simulink model "RLC_model_2_input_finder"  (R2022a)
settings: Solver=FixedStepAuto  StartTime=0.0  StopTime=.004  FixedStep=1e-7  RelTol=1e-3
model workspace (MAT data in the model file):
  Amplitude = 1800
values from neighbouring files (symbols this model uses):
  Amp = Amplitude    [RLC_input_finder.m]
  frequency = round(double(frequency))    [RLC_Square_Wave_Driver.m]    (also in RLC_input_finder.m = i; Voltage_Waveform_Generator.m = 19000)
libraries: spsSeriesRLCBranchLib x15, spsVoltageMeasurementLib x5, simulink x3, spsControlledVoltageSourceLib x3, spsCurrentMeasurementLib x3, spsParallelRLCBranchLib x3, spsACCurrentSourceLib x1, spspowerguiLib x1
settings Model: Creator=ducks  LastModifiedBy=ducks

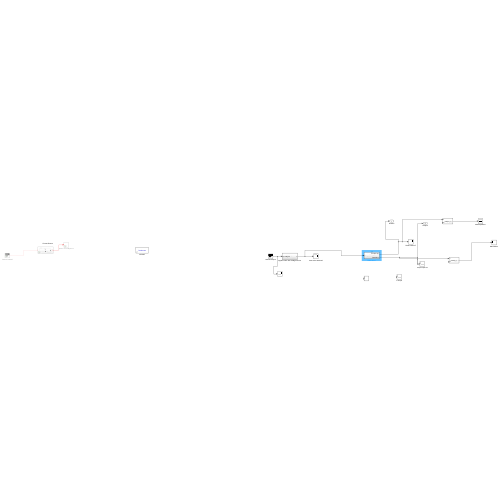
[thumbnail: Simulink's stored preview of the top-level diagram]
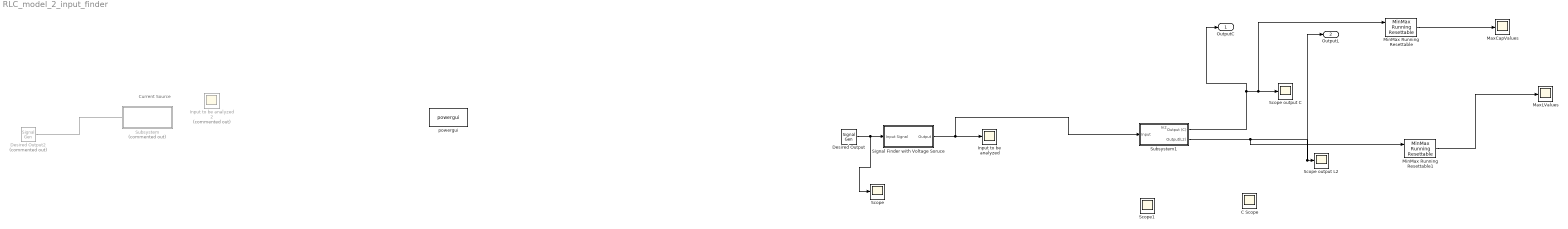
== system RLC_model_2_input_finder ==
  note: Current Source
  C Scope : Scope
  Desired Output : SignalGenerator  Amplitude=Amp  Frequency=frequency
  Desired Output2 : SignalGenerator  Commented=on  Amplitude=10000  Frequency=19100
  Input to be analyzed : Scope
  Input to be analyzed 2 : Scope  Commented=on
  MaxCapValues : Scope
  MaxLValues : Scope
  MinMax Running Resettable : simulink/Math Operations/MinMax Running Resettable  Function=max  vinit=0.0
  MinMax Running Resettable1 : simulink/Math Operations/MinMax Running Resettable  Function=max  vinit=0.0
  Scope : Scope
  Scope output C : Scope
  Scope output L2 : Scope
  Scope1 : Scope
  Signal Finder with Voltage Soruce : Subsystem
  Subsystem : Subsystem  Commented=on
  Subsystem1 : Subsystem
      settings: PortSchema="{\"entries\":[{\"content\":{\"sides\":[{\"content\":{\"connectorIds\":[\"In1\"]},\"type\":\"ConnectorPlacement.EquallySpacedRectSide\",\"uuid\":\"875611cf-7eb9-4d9d-822a-bd3f6d836b83\"},{\"content\":{\"connectorIds\":[\"Out1\",\"Out2\"],\"side\":\"RIGHT\"},\"type\":\"ConnectorPlacement.EquallySpacedRectSide\",\"uuid\":\"445ca6a9-d919-4b8d-ac4c-5af6ec8f882d\"},{\"content\":{\"connectorIds\":[\"In2\"],\"side\":\"TOP\"},\"type\":\"ConnectorPlacement.EquallySpacedRectSide\",\"uuid\":\"dd4cb797-8dc0-482e-83b9-0fae008e5cb7\"}]},\"type\":\"ConnectorPlacement.EquallySpacedConnector\",\"uuid\":\"ab642c4d-046c-490f-ad99-85f64f30cc72\"}],\"packageUris\":[\"http://schema.mathworks.com/mf0/Connector/R2020b\"],\"version\":\"1.0\"}"
  powergui : spspowerguiLib/powergui  Priority=1  SimulationMode=Continuous  SampleTime=50e-6  frequency=60  Iterations=50  frequencyindice=0  Pbase=100e6  ErrMax=1e-4  UnitsV=kV  UnitsW=MW  buscounter=0  FunctionMessages=off  echomessages=off  EnableUseOfTLC=off  CurrentSourceSwitches=off  DisableSnubberDevices=off  DisableRonSwitches=off  DisableVfSwitches=off  DisplayEquations=off  AutomaticDiscreteSolvers=off  SolverType=Tustin/Backward Euler (TBE)  Interpol=off  ExternalGateDelay=off  methode=off  Ts=100  x0status=blocks  SPID=on  SwTol=0  HookPort=off  NonlinearTolerance=1e-4  nMaxIteration=100  ContinueOnMaxIteration=off  RestoreLinks=warning  ResistiveCurrentMeasurement=off  Frange=[0:2:500]  Ylog=off  Xlog=on  ShowGrid=off  save=off  variable=ZData  structure=0  ZoomFFT=off  StartTime=0.0  cycles=1  DisplayStyle=1  fundamental=60  FreqAxis=off  MaxFrequency=1000  frequencyindicesteady=1  RmsSteady=1  display=off
  OutputC : Outport
  OutputL : Outport  Port=2
  wires:
  Desired Output2/1 -> ?
  ? -> Input to be analyzed 2/1
  Subsystem1/2(Output(L2)) -> MinMax Running Resettable1/1, OutputL/1, Scope output L2/1
  MinMax Running Resettable1/1 -> MaxLValues/1
  Desired Output/1 -> Scope/1, Signal Finder with Voltage Soruce/1(Input Signal)
  MinMax Running Resettable/1 -> MaxCapValues/1
  Subsystem1/1(Output (C)) -> OutputC/1, MinMax Running Resettable/1, Scope output C/1
  Signal Finder with Voltage Soruce/1(Output) -> Subsystem1/1(Input), Input to be analyzed/1

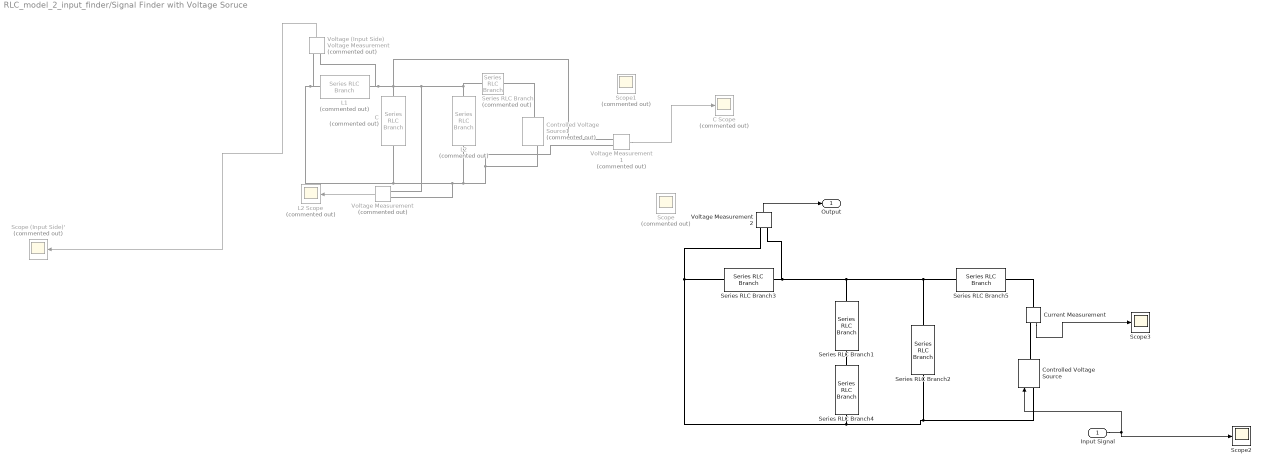
== system RLC_model_2_input_finder/Signal Finder with Voltage Soruce ==
  Input Signal : Inport
  C : spsSeriesRLCBranchLib/Series RLC Branch  Commented=on  LConnTagsString=__new0  RConnTagsString=__new0  BranchType=C  Resistance=1  Inductance=1e-3  SetiL0=off  InitialCurrent=0  Capacitance=96e-6  Setx0=off  InitialVoltage=0  Measurements=None
  C Scope : Scope  Commented=on
  Controlled Voltage Source : spsControlledVoltageSourceLib/Controlled Voltage Source  Initialize=on  Source_Type=AC  Amplitude=0  Phase=0  Frequency=0  Measurements=None
  Controlled Voltage Source1 : spsControlledVoltageSourceLib/Controlled Voltage Source  Commented=on  Initialize=on  Source_Type=DC  Amplitude=5  Phase=0  Frequency=0  Measurements=None
  Current Measurement : spsCurrentMeasurementLib/Current Measurement  PhasorSimulation=off  OutputType=Complex  PSBequivalent=0
  L1 : spsSeriesRLCBranchLib/Series RLC Branch  Commented=on  LConnTagsString=__new0  RConnTagsString=__new0  BranchType=L  Resistance=1  Inductance=1.4e-6  SetiL0=off  InitialCurrent=0  Capacitance=0  Setx0=off  InitialVoltage=0  Measurements=None
  L2 : spsSeriesRLCBranchLib/Series RLC Branch  Commented=on  LConnTagsString=__new0  RConnTagsString=__new0  BranchType=L  Resistance=1  Inductance=1.5e-6  SetiL0=off  InitialCurrent=0  Capacitance=1e-6  Setx0=off  InitialVoltage=0  Measurements=None
  L2 Scope : Scope  Commented=on
  Scope : Scope  Commented=on
  Scope (Input Side)' : Scope  Commented=on
  Scope1 : Scope  Commented=on
  Scope2 : Scope
  Scope3 : Scope
  Series RLC Branch : spsSeriesRLCBranchLib/Series RLC Branch  Commented=on  LConnTagsString=__new0  RConnTagsString=__new0  BranchType=R  Resistance=.001  Inductance=1e-3  SetiL0=off  InitialCurrent=0  Capacitance=1e-6  Setx0=off  InitialVoltage=0  Measurements=None
  Series RLC Branch1 : spsSeriesRLCBranchLib/Series RLC Branch  LConnTagsString=__new0  RConnTagsString=__new0  BranchType=C  Resistance=1  Inductance=1e-3  SetiL0=off  InitialCurrent=0  Capacitance=96e-6  Setx0=off  InitialVoltage=0  Measurements=None
  Series RLC Branch2 : spsSeriesRLCBranchLib/Series RLC Branch  LConnTagsString=__new0  RConnTagsString=__new0  BranchType=L  Resistance=1  Inductance=1.5e-6  SetiL0=off  InitialCurrent=0  Capacitance=1e-6  Setx0=off  InitialVoltage=0  Measurements=None
  Series RLC Branch3 : spsSeriesRLCBranchLib/Series RLC Branch  LConnTagsString=__new0  RConnTagsString=__new0  BranchType=L  Resistance=1  Inductance=1.4e-6  SetiL0=off  InitialCurrent=0  Capacitance=1e-6  Setx0=off  InitialVoltage=0  Measurements=None
  Series RLC Branch4 : spsSeriesRLCBranchLib/Series RLC Branch  LConnTagsString=__new0  RConnTagsString=__new0  BranchType=R  Resistance=.00159  Inductance=1e-3  SetiL0=off  InitialCurrent=0  Capacitance=1e-6  Setx0=off  InitialVoltage=0  Measurements=None
  Series RLC Branch5 : spsSeriesRLCBranchLib/Series RLC Branch  LConnTagsString=__new0  RConnTagsString=__new0  BranchType=R  Resistance=.01  Inductance=1e-3  SetiL0=off  InitialCurrent=0  Capacitance=1e-6  Setx0=off  InitialVoltage=0  Measurements=None
  Voltage (Input Side) : spsVoltageMeasurementLib/Voltage Measurement  Commented=on  PhasorSimulation=off  OutputType=Complex  PSBequivalent=0
  Voltage Measurement : spsVoltageMeasurementLib/Voltage Measurement  Commented=on  PhasorSimulation=off  OutputType=Complex  PSBequivalent=0
  Voltage Measurement1 : spsVoltageMeasurementLib/Voltage Measurement  Commented=on  PhasorSimulation=off  OutputType=Complex  PSBequivalent=0
  Voltage Measurement2 : spsVoltageMeasurementLib/Voltage Measurement  PhasorSimulation=off  OutputType=Complex  PSBequivalent=0
  Output : Outport
  wires:
  Voltage Measurement/1 -> L2 Scope/1
  Voltage (Input Side)/1 -> Scope (Input Side)'/1
  Voltage Measurement1/1 -> C Scope/1
  Input Signal/1 -> Controlled Voltage Source/1, Scope2/1
  Current Measurement/1 -> Scope3/1
  Voltage Measurement2/1 -> Output/1
  connections:
  Voltage Measurement1/LConn1 -- Series RLC Branch/LConn1 -- L2/LConn1 -- Voltage Measurement/LConn2 -- Voltage (Input Side)/LConn2 -- L1/RConn1 -- C/LConn1
  Controlled Voltage Source1/LConn1 -- Voltage Measurement1/LConn2 -- L2/RConn1 -- C/RConn1 -- Voltage (Input Side)/LConn1 -- L1/LConn1 -- Voltage Measurement/LConn1
  Series RLC Branch/RConn1 -- Controlled Voltage Source1/RConn1
  Controlled Voltage Source/LConn1 -- Series RLC Branch4/RConn1 -- Series RLC Branch3/LConn1 -- Voltage Measurement2/LConn1 -- Series RLC Branch2/RConn1
  Current Measurement/RConn1 -- Controlled Voltage Source/RConn1
  Series RLC Branch3/RConn1 -- Series RLC Branch5/LConn1 -- Series RLC Branch2/LConn1 -- Series RLC Branch1/LConn1 -- Voltage Measurement2/LConn2
  Series RLC Branch4/LConn1 -- Series RLC Branch1/RConn1
  Series RLC Branch5/RConn1 -- Current Measurement/LConn1

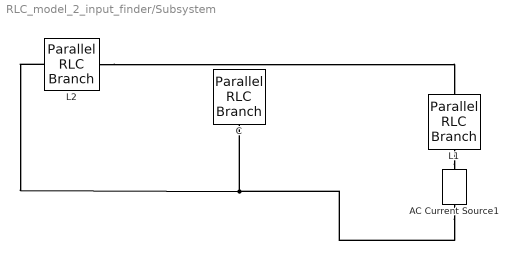
== system RLC_model_2_input_finder/Subsystem ==
  AC Current Source1 : spsACCurrentSourceLib/AC Current Source  Amplitude=1800  Phase=0  Frequency=19500  SampleTime=0  Measurements=None
      settings: SourceProductBaseCode=PS
  C : spsParallelRLCBranchLib/Parallel RLC Branch  LConnTagsString=a  RConnTagsString=__new0  BranchType=C  Resistance=1  Inductance=1e-3  SetiL0=off  InitialCurrent=0  Capacitance=96e-6  Setx0=off  InitialVoltage=0  Measurements=None
  L1 : spsParallelRLCBranchLib/Parallel RLC Branch  LConnTagsString=a  RConnTagsString=__new0  BranchType=L  Resistance=1  Inductance=2e-6  SetiL0=off  InitialCurrent=0  Capacitance=1e-6  Setx0=off  InitialVoltage=0  Measurements=None
  L2 : spsParallelRLCBranchLib/Parallel RLC Branch  LConnTagsString=a  RConnTagsString=__new0  BranchType=L  Resistance=1  Inductance=10e-6  SetiL0=off  InitialCurrent=0  Capacitance=1e-6  Setx0=off  InitialVoltage=0  Measurements=None
  connections:
  L2/RConn1 -- L1/LConn1
  L1/RConn1 -- AC Current Source1/RConn1
  AC Current Source1/LConn1 -- C/RConn1 -- L2/LConn1

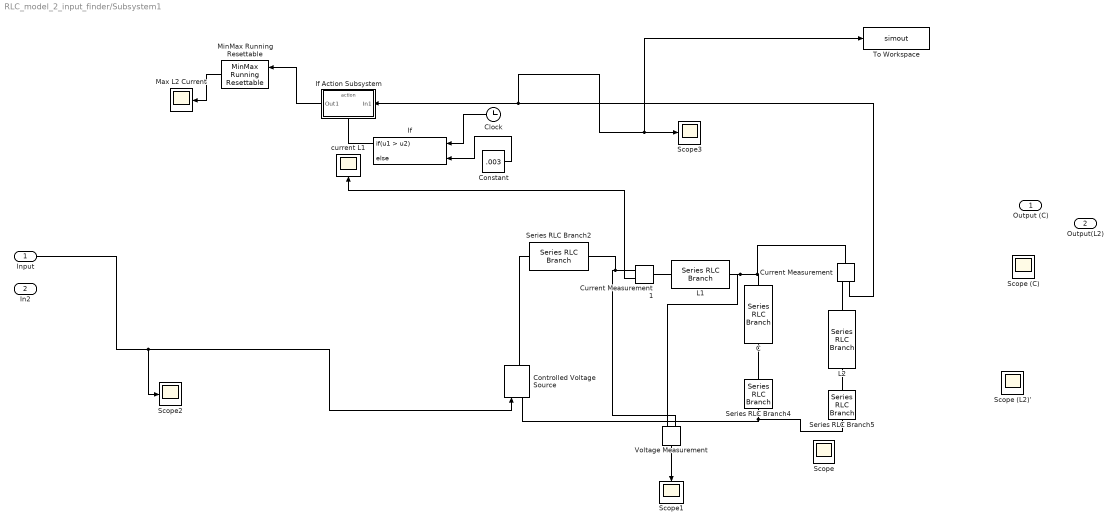
== system RLC_model_2_input_finder/Subsystem1 ==
  Input : Inport
  In2 : Inport  Port=2
  C : spsSeriesRLCBranchLib/Series RLC Branch  LConnTagsString=__new0  RConnTagsString=__new0  BranchType=C  Resistance=1  Inductance=1e-3  SetiL0=off  InitialCurrent=0  Capacitance=96e-6  Setx0=off  InitialVoltage=0  Measurements=None
  Clock : Clock
  Constant : Constant  Value=.003
  Controlled Voltage Source : spsControlledVoltageSourceLib/Controlled Voltage Source  Initialize=on  Source_Type=AC  Amplitude=0  Phase=0  Frequency=0  Measurements=None
  Current Measurement : spsCurrentMeasurementLib/Current Measurement  PhasorSimulation=off  OutputType=Complex  PSBequivalent=0
  Current Measurement1 : spsCurrentMeasurementLib/Current Measurement  PhasorSimulation=off  OutputType=Complex  PSBequivalent=0
  If : If  NumInputs=2  IfExpression=u1 > u2
  If Action Subsystem : Subsystem  TreatAsAtomicUnit=on
  L1 : spsSeriesRLCBranchLib/Series RLC Branch  LConnTagsString=__new0  RConnTagsString=__new0  BranchType=L  Resistance=1  Inductance=1.4e-6  SetiL0=off  InitialCurrent=0  Capacitance=0  Setx0=off  InitialVoltage=0  Measurements=None
  L2 : spsSeriesRLCBranchLib/Series RLC Branch  LConnTagsString=__new0  RConnTagsString=__new0  BranchType=L  Resistance=1  Inductance=1.5e-6  SetiL0=off  InitialCurrent=0  Capacitance=1e-6  Setx0=off  InitialVoltage=0  Measurements=None
  Max L2 Current : Scope
  MinMax Running Resettable : simulink/Math Operations/MinMax Running Resettable  Function=max  vinit=0.0
  Scope{,1..3} (4 alike) : Scope
  Scope (C) : Scope
  Scope (L2)' : Scope
  Series RLC Branch2 : spsSeriesRLCBranchLib/Series RLC Branch  LConnTagsString=__new0  RConnTagsString=__new0  BranchType=R  Resistance=.00164  Inductance=1e-3  SetiL0=off  InitialCurrent=0  Capacitance=1e-6  Setx0=off  InitialVoltage=0  Measurements=None
  Series RLC Branch4 : spsSeriesRLCBranchLib/Series RLC Branch  LConnTagsString=__new0  RConnTagsString=__new0  BranchType=R  Resistance=.00205  Inductance=1e-3  SetiL0=off  InitialCurrent=0  Capacitance=1e-6  Setx0=off  InitialVoltage=0  Measurements=None
  Series RLC Branch5 : spsSeriesRLCBranchLib/Series RLC Branch  LConnTagsString=__new0  RConnTagsString=__new0  BranchType=R  Resistance=.00205  Inductance=1e-3  SetiL0=off  InitialCurrent=0  Capacitance=1e-6  Setx0=off  InitialVoltage=0  Measurements=None
  To Workspace : ToWorkspace  VariableName=simout  SaveFormat=Timeseries  SampleTime=-1
  Voltage Measurement : spsVoltageMeasurementLib/Voltage Measurement  PhasorSimulation=off  OutputType=Complex  PSBequivalent=0
  current L1 : Scope
  Output (C) : Outport
  Output(L2) : Outport  Port=2
  wires:
  Voltage Measurement/1 -> Scope1/1
  Input/1 -> Scope2/1, Controlled Voltage Source/1
  Current Measurement/1 -> If Action Subsystem/1(In1), To Workspace/1, Scope3/1
  Current Measurement1/1 -> current L1/1
  Clock/1 -> If/1
  Constant/1 -> If/2
  If/1 -> If Action Subsystem/Action
  If Action Subsystem/1(Out1) -> MinMax Running Resettable/1
  MinMax Running Resettable/1 -> Max L2 Current/1
  connections:
  Current Measurement1/RConn1 -- Series RLC Branch2/LConn1 -- Voltage Measurement/LConn1
  L2/LConn1 -- Current Measurement/RConn1
  L1/LConn1 -- Current Measurement1/LConn1
  Series RLC Branch4/RConn1 -- Series RLC Branch5/RConn1 -- Controlled Voltage Source/LConn1
  Voltage Measurement/LConn2 -- L1/RConn1 -- Current Measurement/LConn1 -- C/LConn1
  Series RLC Branch2/RConn1 -- Controlled Voltage Source/RConn1
  Series RLC Branch4/LConn1 -- C/RConn1
  Series RLC Branch5/LConn1 -- L2/RConn1

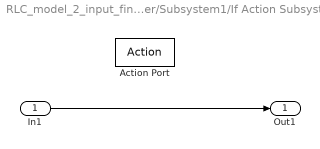
== system RLC_model_2_input_finder/Subsystem1/If Action Subsystem ==
  In1 : Inport
  Action Port : ActionPort  ActionPortLabel=if(u1 > u2)
  Out1 : Outport
  wires:
  In1/1 -> Out1/1
